simulink model "testbench_model_2019a"  (R2019a)
settings: Solver=ode15s  StartTime=0.0  StopTime=tsim  RelTol=1e-3  EnableMultiTasking=on
values from neighbouring files (symbols this model uses):
  a = randn(1,5)    [magnetic_dist_noise.m]    (also in matlab.mat = 1000)
  g = 9.81    [matlab.mat]    (also in system_dynamics.m = evalin('base','g'))
  Kd1 = 55255.4666667    [matlab.mat]
  Kd3 = 22055.4666667    [matlab.mat]
  Kd4 = 0.01059999556    [matlab.mat]
  Ki1 = 1786382.33784    [matlab.mat]
  Ki3 = 714981.495471    [matlab.mat]
  Ki4 = 13.0608621147    [matlab.mat]
  Kp1 = 551410.490045    [matlab.mat]
  Kp3 = 220696.481621    [matlab.mat]
  Kp4 = 0.623941757147    [matlab.mat]
  mb = 0.2    [matlab.mat]    (also in system_dynamics.m = evalin('base','mb'))
  mj3 = 200    [matlab.mat]    (also in system_dynamics.m = evalin('base','mj3'))
  Tsampling = 0.01    [matlab.mat]
libraries: simulink x9, aerolibnav x2
settings Model: Creator=Akos  LastModifiedBy=akosodry
settings DataIOCC: LimitDataPoints=on  SaveFormat=Array  ReturnWorkspaceOutputs=off
settings OptimizationCC: LifeSpan=inf
settings DebuggingCC: SFUnexpectedBacktrackingDiag=warning  SFNoUnconditionalDefaultTransitionDiag=warning  SFExecutionAtInitializationDiag=none  ArithmeticOperatorsInVariantConditions=warning
settings HardwareCC: ProdBitPerPointer=32  ProdBitPerSizeT=32  ProdBitPerPtrDiffT=32  ProdLargestAtomicFloat=None  ProdIntDivRoundTo=Undefined  ProdEndianess=Unspecified  ProdWordSize=32  ProdHWDeviceType=32-bit Generic
settings ModelReferenceCC: PropagateSignalLabelsOutOfModel=off
settings SFSimCC: SimUseLocalCustomCode=off
settings RTWCC: RTWUseLocalCustomCode=off
settings CodeAppCC: StateflowObjectComments=on
settings GRTTargetCC: TargetLangStandard=C89/C90 (ANSI)  GeneratePreprocessorConditionals=Disable all
settings ConfigComp: CovMetricSettings=dw  CovHtmlReporting=on  CovSaveCumulativeToWorkspaceVar=on  CovSaveSingleToWorkspaceVar=on  CovExternalEMLEnable=off

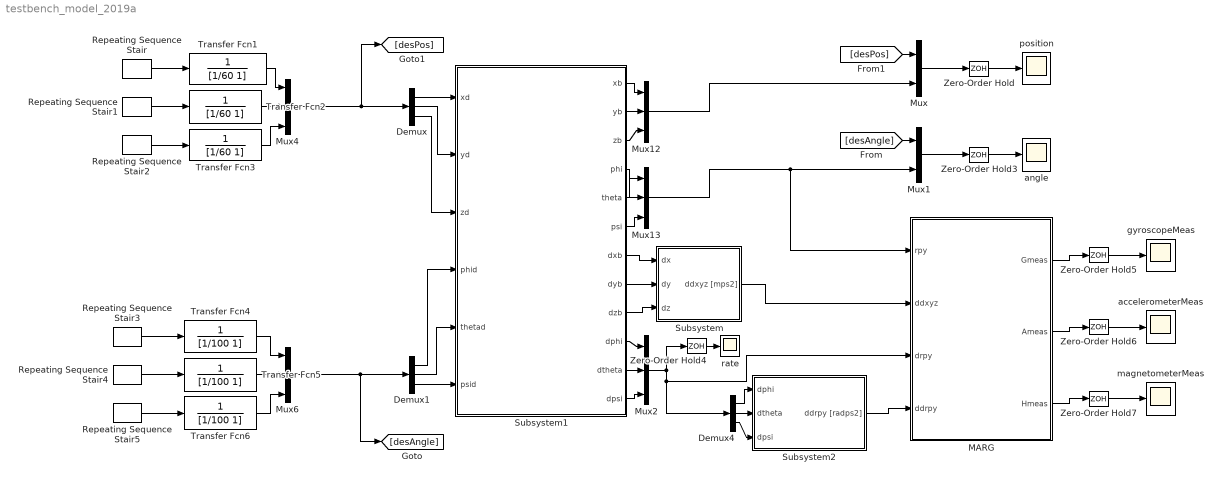
== system testbench_model_2019a ==
  Demux : Demux  Outputs=3
  Demux1 : Demux  Outputs=3
  Demux4 : Demux  Outputs=3
  MARG : Subsystem
  Mux : Mux  Inputs=2
  Mux1 : Mux  Inputs=2
  Mux{2,4,6,12..13} (5 alike) : Mux  Inputs=3
  Repeating Sequence Stair : simulink/Sources/Repeating Sequence Stair  OutValues=[0.5 0.4 0.5 0.1 0.05 0.1 0.9 0.8 0.9].'  tsamp=0.25  OutMin=[]  OutMax=[]  OutDataTypeStr=double  OutputDataTypeScalingMode=double  OutDataType=fixdt(0,8)  ConRadixGroup=Best Precision: Vector-wise  OutScaling=2^-12
  Repeating Sequence Stair1 : simulink/Sources/Repeating Sequence Stair  OutValues=[0.2 0.3 0.2 0.8 0.7 0.8 0.4 0.5 0.4].'  tsamp=0.25  OutMin=[]  OutMax=[]  OutDataTypeStr=double  OutputDataTypeScalingMode=double  OutDataType=fixdt(0,8)  ConRadixGroup=Best Precision: Vector-wise  OutScaling=2^-12
  Repeating Sequence Stair2 : simulink/Sources/Repeating Sequence Stair  OutValues=[0.3 0.2 0.3 0 0.1 0 0.51 0.61 0.51].'  tsamp=0.25  OutMin=[]  OutMax=[]  OutDataTypeStr=double  OutputDataTypeScalingMode=double  OutDataType=fixdt(0,8)  ConRadixGroup=Best Precision: Vector-wise  OutScaling=2^-12
  Repeating Sequence Stair3 : simulink/Sources/Repeating Sequence Stair  OutValues=[0 0.1 0 0.75 0.85 0.75 -0.57 -0.47 -0.57].'  tsamp=0.25  OutMin=[]  OutMax=[]  OutDataTypeStr=double  OutputDataTypeScalingMode=double  OutDataType=fixdt(0,8)  ConRadixGroup=Best Precision: Vector-wise  OutScaling=2^-12
  Repeating Sequence Stair4 : simulink/Sources/Repeating Sequence Stair  OutValues=[0 -0.1 0 0.75 0.65 0.75 -0.19 -0.29 -0.19].'  tsamp=0.25  OutMin=[]  OutMax=[]  OutDataTypeStr=double  OutputDataTypeScalingMode=double  OutDataType=fixdt(0,8)  ConRadixGroup=Best Precision: Vector-wise  OutScaling=2^-12
  Repeating Sequence Stair5 : simulink/Sources/Repeating Sequence Stair  OutValues=[0 0.1 0.1 0.75 0.6 0.75 0.38 0.5 0.38].'  tsamp=0.25  OutMin=[]  OutMax=[]  OutDataTypeStr=double  OutputDataTypeScalingMode=double  OutDataType=fixdt(0,8)  ConRadixGroup=Best Precision: Vector-wise  OutScaling=2^-12
  Subsystem : Subsystem
  Subsystem1 : Subsystem
  Subsystem2 : Subsystem
  Transfer Fcn1 : TransferFcn  Denominator=[1/60 1]
  Transfer Fcn2 : TransferFcn  Denominator=[1/60 1]
  Transfer Fcn3 : TransferFcn  Denominator=[1/60 1]
  Transfer Fcn4 : TransferFcn  Denominator=[1/100 1]
  Transfer Fcn5 : TransferFcn  Denominator=[1/100 1]
  Transfer Fcn6 : TransferFcn  Denominator=[1/100 1]
  Zero-Order Hold{,3..7} (6 alike) : ZeroOrderHold  SampleTime=Tsampling
  accelerometerMeas : Scope
  angle : Scope
  gyroscopeMeas : Scope
  magnetometerMeas : Scope
  position : Scope
  rate : Scope
  wires:
  Mux/1 -> Zero-Order Hold/1
  Mux2/1 -> Demux4/1, MARG/3(drpy), Zero-Order Hold4/1
  Subsystem1/7(dxb) -> Subsystem/1(dx)
  Subsystem1/8(dyb) -> Subsystem/2(dy)
  Subsystem1/9(dzb) -> Subsystem/3(dz)
  Subsystem1/10(dphi) -> Mux2/1
  Subsystem1/11(dtheta) -> Mux2/2
  Subsystem1/12(dpsi) -> Mux2/3
  Repeating Sequence Stair1/1 -> Transfer Fcn2/1
  Repeating Sequence Stair/1 -> Transfer Fcn1/1
  Repeating Sequence Stair2/1 -> Transfer Fcn3/1
  Mux4/1 -> [desPos], Demux/1
  Demux/1 -> Subsystem1/1(xd)
  Demux/2 -> Subsystem1/2(yd)
  Demux/3 -> Subsystem1/3(zd)
  Mux6/1 -> [desAngle], Demux1/1
  Demux1/3 -> Subsystem1/6(psid)
  Demux1/2 -> Subsystem1/5(thetad)
  Demux1/1 -> Subsystem1/4(phid)
  [desAngle] -> Mux1/1
  [desPos] -> Mux/1
  Repeating Sequence Stair4/1 -> Transfer Fcn5/1
  Repeating Sequence Stair3/1 -> Transfer Fcn4/1
  Repeating Sequence Stair5/1 -> Transfer Fcn6/1
  Mux1/1 -> Zero-Order Hold3/1
  Zero-Order Hold/1 -> position/1
  Zero-Order Hold3/1 -> angle/1
  Zero-Order Hold4/1 -> rate/1
  Subsystem1/2(yb) -> Mux12/2
  Subsystem1/3(zb) -> Mux12/3
  Subsystem1/1(xb) -> Mux12/1
  Mux12/1 -> Mux/2
  Subsystem1/4(phi) -> Mux13/1
  Subsystem1/5(theta) -> Mux13/2
  Subsystem1/6(psi) -> Mux13/3
  Mux13/1 -> MARG/1(rpy), Mux1/2
  Demux4/2 -> Subsystem2/2(dtheta)
  Demux4/1 -> Subsystem2/1(dphi)
  Demux4/3 -> Subsystem2/3(dpsi)
  Subsystem/1(ddxyz [mps2]) -> MARG/2(ddxyz)
  Subsystem2/1(ddrpy [radps2]) -> MARG/4(ddrpy)
  MARG/1(Gmeas) -> Zero-Order Hold5/1
  MARG/2(Ameas) -> Zero-Order Hold6/1
  MARG/3(Hmeas) -> Zero-Order Hold7/1
  Transfer Fcn1/1 -> Mux4/1
  Transfer Fcn2/1 -> Mux4/2
  Transfer Fcn3/1 -> Mux4/3
  Transfer Fcn4/1 -> Mux6/1
  Transfer Fcn5/1 -> Mux6/2
  Transfer Fcn6/1 -> Mux6/3
  Zero-Order Hold5/1 -> gyroscopeMeas/1
  Zero-Order Hold6/1 -> accelerometerMeas/1
  Zero-Order Hold7/1 -> magnetometerMeas/1

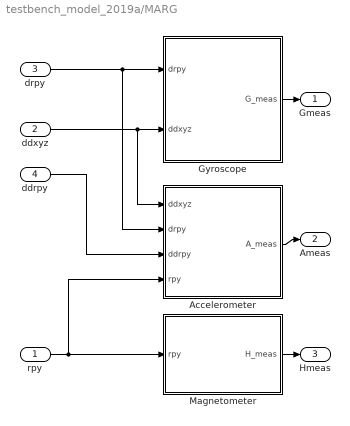
== system testbench_model_2019a/MARG ==
  rpy : Inport
  ddxyz : Inport  Port=2
  drpy : Inport  Port=3
  ddrpy : Inport  Port=4
  Accelerometer : Subsystem
  Gyroscope : Subsystem
  Magnetometer : Subsystem
  Gmeas : Outport
  Ameas : Outport  Port=2
  Hmeas : Outport  Port=3
  wires:
  Magnetometer/1(H_meas) -> Hmeas/1
  Accelerometer/1(A_meas) -> Ameas/1
  Gyroscope/1(G_meas) -> Gmeas/1
  drpy/1 -> Accelerometer/2(drpy), Gyroscope/1(drpy)
  ddrpy/1 -> Accelerometer/3(ddrpy)
  rpy/1 -> Accelerometer/4(rpy), Magnetometer/1(rpy)
  ddxyz/1 -> Gyroscope/2(ddxyz), Accelerometer/1(ddxyz)

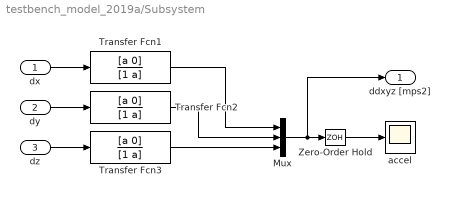
== system testbench_model_2019a/Subsystem ==
  dx : Inport
  dy : Inport  Port=2
  dz : Inport  Port=3
  Mux : Mux  Inputs=3
  Transfer Fcn1 : TransferFcn  Numerator=[a 0]  Denominator=[1 a]
  Transfer Fcn2 : TransferFcn  Numerator=[a 0]  Denominator=[1 a]
  Transfer Fcn3 : TransferFcn  Numerator=[a 0]  Denominator=[1 a]
  Zero-Order Hold : ZeroOrderHold  SampleTime=Tsampling
  accel : Scope
  ddxyz [mps2] : Outport
  wires:
  dz/1 -> Transfer Fcn3/1
  dx/1 -> Transfer Fcn1/1
  dy/1 -> Transfer Fcn2/1
  Transfer Fcn1/1 -> Mux/1
  Mux/1 -> ddxyz [mps2]/1, Zero-Order Hold/1
  Transfer Fcn2/1 -> Mux/2
  Transfer Fcn3/1 -> Mux/3
  Zero-Order Hold/1 -> accel/1

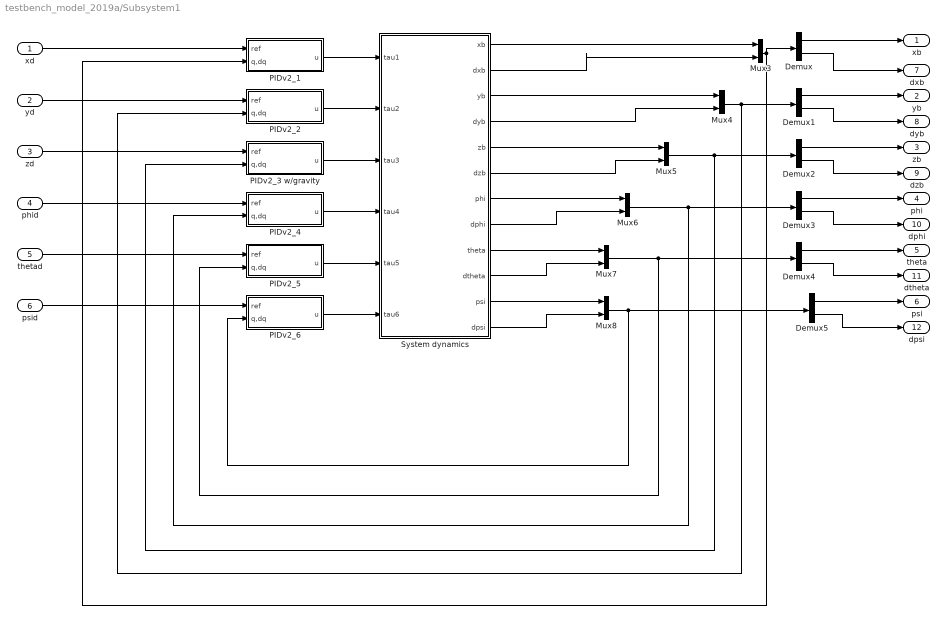
== system testbench_model_2019a/Subsystem1 ==
  xd : Inport
  yd : Inport  Port=2
  zd : Inport  Port=3
  phid : Inport  Port=4
  thetad : Inport  Port=5
  psid : Inport  Port=6
  Demux{,1..5} (6 alike) : Demux  Outputs=2
  Mux{3..8} (6 alike) : Mux  Inputs=2
  PIDv2_1 : Subsystem
  PIDv2_2 : Subsystem
  PIDv2_3 w/gravity : Subsystem
  PIDv2_4 : Subsystem
  PIDv2_5 : Subsystem
  PIDv2_6 : Subsystem
  System dynamics : Subsystem
  xb : Outport
  yb : Outport  Port=2
  zb : Outport  Port=3
  phi : Outport  Port=4
  theta : Outport  Port=5
  psi : Outport  Port=6
  dxb : Outport  Port=7
  dyb : Outport  Port=8
  dzb : Outport  Port=9
  dphi : Outport  Port=10
  dtheta : Outport  Port=11
  dpsi : Outport  Port=12
  wires:
  PIDv2_5/1(u) -> System dynamics/5(tau5)
  Mux3/1 -> Demux/1, PIDv2_1/2(q,dq)
  Demux1/2 -> dyb/1
  Mux8/1 -> Demux5/1, PIDv2_6/2(q,dq)
  Demux4/1 -> theta/1
  psid/1 -> PIDv2_6/1(ref)
  yd/1 -> PIDv2_2/1(ref)
  Mux5/1 -> Demux2/1, PIDv2_3 w/gravity/2(q,dq)
  Demux2/2 -> dzb/1
  xd/1 -> PIDv2_1/1(ref)
  Demux3/1 -> phi/1
  PIDv2_2/1(u) -> System dynamics/2(tau2)
  System dynamics/9(theta) -> Mux7/1
  Demux/1 -> xb/1
  Mux4/1 -> Demux1/1, PIDv2_2/2(q,dq)
  Demux/2 -> dxb/1
  Demux5/2 -> dpsi/1
  System dynamics/12(dpsi) -> Mux8/2
  Mux7/1 -> Demux4/1, PIDv2_5/2(q,dq)
  Mux6/1 -> Demux3/1, PIDv2_4/2(q,dq)
  Demux3/2 -> dphi/1
  phid/1 -> PIDv2_4/1(ref)
  System dynamics/8(dphi) -> Mux6/2
  Demux2/1 -> zb/1
  PIDv2_1/1(u) -> System dynamics/1(tau1)
  Demux1/1 -> yb/1
  System dynamics/3(yb) -> Mux4/1
  PIDv2_4/1(u) -> System dynamics/4(tau4)
  System dynamics/7(phi) -> Mux6/1
  System dynamics/1(xb) -> Mux3/1
  System dynamics/10(dtheta) -> Mux7/2
  System dynamics/6(dzb) -> Mux5/2
  System dynamics/11(psi) -> Mux8/1
  Demux4/2 -> dtheta/1
  PIDv2_6/1(u) -> System dynamics/6(tau6)
  Demux5/1 -> psi/1
  zd/1 -> PIDv2_3 w/gravity/1(ref)
  System dynamics/2(dxb) -> Mux3/2
  System dynamics/4(dyb) -> Mux4/2
  thetad/1 -> PIDv2_5/1(ref)
  PIDv2_3 w/gravity/1(u) -> System dynamics/3(tau3)
  System dynamics/5(zb) -> Mux5/1

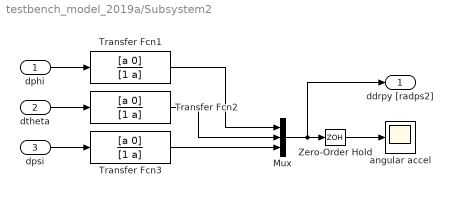
== system testbench_model_2019a/Subsystem2 ==
  dphi : Inport
  dtheta : Inport  Port=2
  dpsi : Inport  Port=3
  Mux : Mux  Inputs=3
  Transfer Fcn1 : TransferFcn  Numerator=[a 0]  Denominator=[1 a]
  Transfer Fcn2 : TransferFcn  Numerator=[a 0]  Denominator=[1 a]
  Transfer Fcn3 : TransferFcn  Numerator=[a 0]  Denominator=[1 a]
  Zero-Order Hold : ZeroOrderHold  SampleTime=Tsampling
  angular accel : Scope
  ddrpy [radps2] : Outport
  wires:
  dpsi/1 -> Transfer Fcn3/1
  dphi/1 -> Transfer Fcn1/1
  dtheta/1 -> Transfer Fcn2/1
  Transfer Fcn1/1 -> Mux/1
  Mux/1 -> ddrpy [radps2]/1, Zero-Order Hold/1
  Transfer Fcn2/1 -> Mux/2
  Transfer Fcn3/1 -> Mux/3
  Zero-Order Hold/1 -> angular accel/1

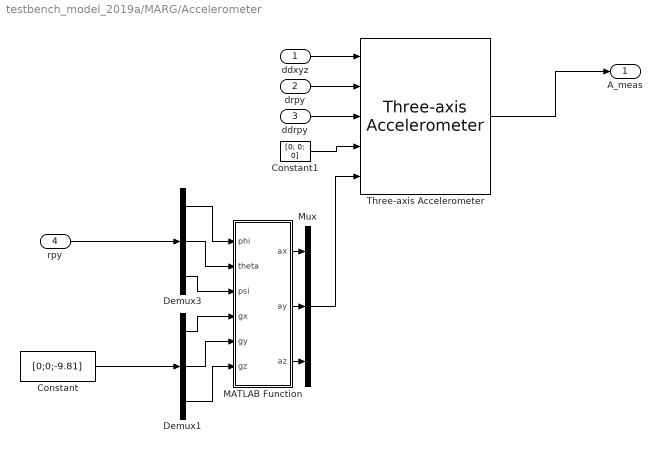
== system testbench_model_2019a/MARG/Accelerometer ==
  ddxyz : Inport
  drpy : Inport  Port=2
  ddrpy : Inport  Port=3
  rpy : Inport  Port=4
  Constant : Constant  Value=[0;0;-9.81]
  Constant1 : Constant  Value=[0; 0; 0]
  Demux1 : Demux  Outputs=3
  Demux3 : Demux  Outputs=3
  MATLAB Function : MATLAB Function  TreatAsAtomicUnit=on
  Mux : Mux  Inputs=3
  Three-axis Accelerometer : aerolibnav/Three-axis Accelerometer  units=Metric (MKS)  acc=[0 0 0]  gtype=on  dtype_a=off  w_a=190  z_a=0.707  a_sf_cc=[1 0 0; 0 1 0; 0 0 1]  a_bias=[0 0 0]  a_Ts=Tsampling  a_rand=on  a_seeds=[23093 23094 23095]  a_pow=[0.0005 0.0005 0.0005]  a_sat="[-inf  -inf  -inf  inf inf inf]"
      settings: SourceProductName=Aerospace Blockset  SourceProductBaseCode=AE
  A_meas : Outport
  wires:
  Three-axis Accelerometer/1 -> A_meas/1
  ddxyz/1 -> Three-axis Accelerometer/1
  Demux1/2 -> MATLAB Function/5(gy)
  Demux3/1 -> MATLAB Function/1(phi)
  Demux3/2 -> MATLAB Function/2(theta)
  MATLAB Function/2(ay) -> Mux/2
  Demux3/3 -> MATLAB Function/3(psi)
  Demux1/3 -> MATLAB Function/6(gz)
  MATLAB Function/1(ax) -> Mux/1
  MATLAB Function/3(az) -> Mux/3
  Demux1/1 -> MATLAB Function/4(gx)
  rpy/1 -> Demux3/1
  Constant/1 -> Demux1/1
  Mux/1 -> Three-axis Accelerometer/5
  drpy/1 -> Three-axis Accelerometer/2
  ddrpy/1 -> Three-axis Accelerometer/3
  Constant1/1 -> Three-axis Accelerometer/4

== system testbench_model_2019a/MARG/Gyroscope ==
  drpy : Inport
  ddxyz : Inport  Port=2
  Gain2 : Gain  Gain=1/g
  Three-axis Gyroscope : aerolibnav/Three-axis Gyroscope  dtype_g=on  w_g=190  z_g=0.707  g_sf_cc=[1 0 0; 0 1 0; 0 0 1]  g_bias=[0 0 0]  g_sen=[0 0 0]  g_Ts=Tsampling  g_rand=on  g_seeds=[23093 23094 23095]  g_pow=[0.0005 0.0005 0.0005]  g_sat="[-inf  -inf  -inf  inf inf inf]"
      settings: SourceProductName=Aerospace Blockset  SourceProductBaseCode=AE
  G_meas : Outport
  wires:
  ddxyz/1 -> Gain2/1
  Gain2/1 -> Three-axis Gyroscope/2
  Three-axis Gyroscope/1 -> G_meas/1
  drpy/1 -> Three-axis Gyroscope/1

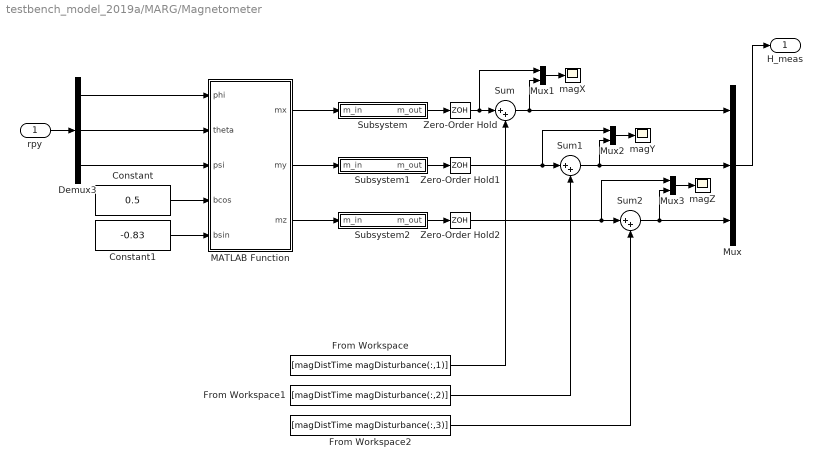
== system testbench_model_2019a/MARG/Magnetometer ==
  rpy : Inport
  Constant : Constant  Value=0.5
  Constant1 : Constant  Value=-0.83
  Demux3 : Demux  Outputs=3
  From Workspace : FromWorkspace  VariableName=[magDistTime magDisturbance(:,1)]  SampleTime=Tsampling
  From Workspace1 : FromWorkspace  VariableName=[magDistTime magDisturbance(:,2)]  SampleTime=Tsampling
  From Workspace2 : FromWorkspace  VariableName=[magDistTime magDisturbance(:,3)]  SampleTime=Tsampling
  MATLAB Function : MATLAB Function  TreatAsAtomicUnit=on
  Mux : Mux  Inputs=3
  Mux1 : Mux  Inputs=2
  Mux2 : Mux  Inputs=2
  Mux3 : Mux  Inputs=2
  Subsystem : Subsystem
  Subsystem1 : Subsystem
  Subsystem2 : Subsystem
  Sum : Sum  Inputs=|++
  Sum1 : Sum  Inputs=|++
  Sum2 : Sum  Inputs=|++
  Zero-Order Hold : ZeroOrderHold  SampleTime=Tsampling
  Zero-Order Hold1 : ZeroOrderHold  SampleTime=Tsampling
  Zero-Order Hold2 : ZeroOrderHold  SampleTime=Tsampling
  magX : Scope
  magY : Scope
  magZ : Scope
  H_meas : Outport
  wires:
  Demux3/3 -> MATLAB Function/3(psi)
  Demux3/1 -> MATLAB Function/1(phi)
  Mux/1 -> H_meas/1
  Constant/1 -> MATLAB Function/4(bcos)
  Constant1/1 -> MATLAB Function/5(bsin)
  MATLAB Function/1(mx) -> Subsystem/1(m_in)
  Subsystem/1(m_out) -> Zero-Order Hold/1
  rpy/1 -> Demux3/1
  Demux3/2 -> MATLAB Function/2(theta)
  MATLAB Function/2(my) -> Subsystem1/1(m_in)
  Subsystem1/1(m_out) -> Zero-Order Hold1/1
  MATLAB Function/3(mz) -> Subsystem2/1(m_in)
  Subsystem2/1(m_out) -> Zero-Order Hold2/1
  Zero-Order Hold/1 -> Mux1/1, Sum/1
  Sum/1 -> Mux1/2, Mux/1
  Zero-Order Hold1/1 -> Mux2/1, Sum1/1
  Sum1/1 -> Mux2/2, Mux/2
  From Workspace/1 -> Sum/2
  Mux1/1 -> magX/1
  From Workspace1/1 -> Sum1/2
  Mux2/1 -> magY/1
  Mux3/1 -> magZ/1
  Sum2/1 -> Mux3/2, Mux/3
  Zero-Order Hold2/1 -> Mux3/1, Sum2/1
  From Workspace2/1 -> Sum2/2

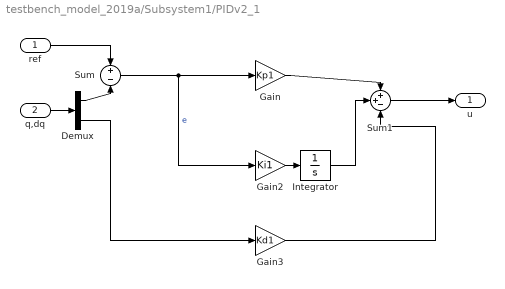
== system testbench_model_2019a/Subsystem1/PIDv2_1 ==
  ref : Inport
  q,dq : Inport  Port=2
  Demux : Demux  Outputs=2
  Gain : Gain  Gain=Kp1
  Gain2 : Gain  Gain=Ki1
  Gain3 : Gain  Gain=Kd1
  Integrator : Integrator
  Sum : Sum  Inputs=+-
  Sum1 : Sum  Inputs=++-
  u : Outport
  wires:
  Sum1/1 -> u/1
  Gain3/1 -> Sum1/3
  Demux/1 -> Sum/2
  Gain2/1 -> Integrator/1
  Gain/1 -> Sum1/1
  Integrator/1 -> Sum1/2
  Demux/2 -> Gain3/1
  q,dq/1 -> Demux/1
  ref/1 -> Sum/1
  Sum/1 -> Gain2/1, Gain/1  "e"

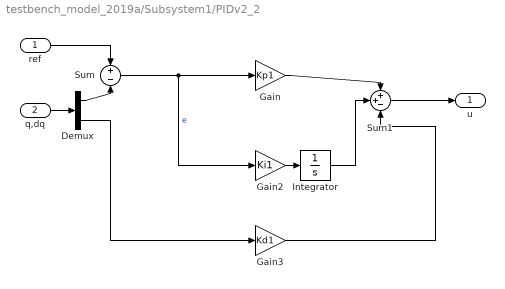
== system testbench_model_2019a/Subsystem1/PIDv2_2 ==
  ref : Inport
  q,dq : Inport  Port=2
  Demux : Demux  Outputs=2
  Gain : Gain  Gain=Kp1
  Gain2 : Gain  Gain=Ki1
  Gain3 : Gain  Gain=Kd1
  Integrator : Integrator
  Sum : Sum  Inputs=+-
  Sum1 : Sum  Inputs=++-
  u : Outport
  wires:
  Sum1/1 -> u/1
  Gain3/1 -> Sum1/3
  Demux/1 -> Sum/2
  Gain2/1 -> Integrator/1
  Gain/1 -> Sum1/1
  Integrator/1 -> Sum1/2
  Demux/2 -> Gain3/1
  q,dq/1 -> Demux/1
  ref/1 -> Sum/1
  Sum/1 -> Gain2/1, Gain/1  "e"

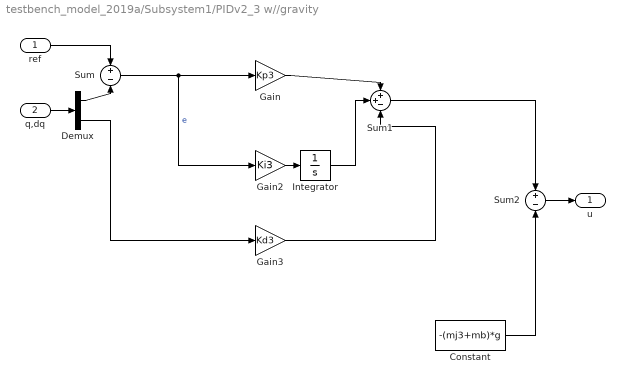
== system testbench_model_2019a/Subsystem1/PIDv2_3 w//gravity ==
  ref : Inport
  q,dq : Inport  Port=2
  Constant : Constant  Value=-(mj3+mb)*g
  Demux : Demux  Outputs=2
  Gain : Gain  Gain=Kp3
  Gain2 : Gain  Gain=Ki3
  Gain3 : Gain  Gain=Kd3
  Integrator : Integrator
  Sum : Sum  Inputs=+-
  Sum1 : Sum  Inputs=++-
  Sum2 : Sum  Inputs=+-
  u : Outport
  wires:
  Gain3/1 -> Sum1/3
  Demux/1 -> Sum/2
  Gain2/1 -> Integrator/1
  Gain/1 -> Sum1/1
  Integrator/1 -> Sum1/2
  Demux/2 -> Gain3/1
  q,dq/1 -> Demux/1
  ref/1 -> Sum/1
  Sum/1 -> Gain2/1, Gain/1  "e"
  Sum1/1 -> Sum2/1
  Constant/1 -> Sum2/2
  Sum2/1 -> u/1

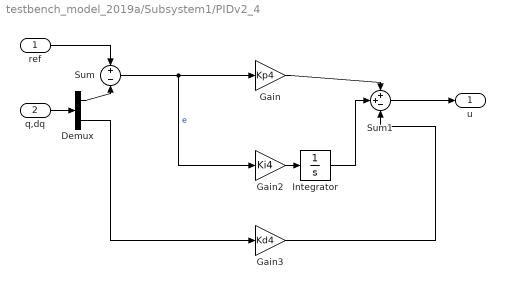
== system testbench_model_2019a/Subsystem1/PIDv2_4 ==
  ref : Inport
  q,dq : Inport  Port=2
  Demux : Demux  Outputs=2
  Gain : Gain  Gain=Kp4
  Gain2 : Gain  Gain=Ki4
  Gain3 : Gain  Gain=Kd4
  Integrator : Integrator
  Sum : Sum  Inputs=+-
  Sum1 : Sum  Inputs=++-
  u : Outport
  wires:
  Sum1/1 -> u/1
  Gain3/1 -> Sum1/3
  Demux/1 -> Sum/2
  Gain2/1 -> Integrator/1
  Gain/1 -> Sum1/1
  Integrator/1 -> Sum1/2
  Demux/2 -> Gain3/1
  q,dq/1 -> Demux/1
  ref/1 -> Sum/1
  Sum/1 -> Gain2/1, Gain/1  "e"

== system testbench_model_2019a/Subsystem1/PIDv2_5 ==
  ref : Inport
  q,dq : Inport  Port=2
  Demux : Demux  Outputs=2
  Gain : Gain  Gain=Kp4
  Gain2 : Gain  Gain=Ki4
  Gain3 : Gain  Gain=Kd4
  Integrator : Integrator
  Sum : Sum  Inputs=+-
  Sum1 : Sum  Inputs=++-
  u : Outport
  wires:
  Sum1/1 -> u/1
  Gain3/1 -> Sum1/3
  Demux/1 -> Sum/2
  Gain2/1 -> Integrator/1
  Gain/1 -> Sum1/1
  Integrator/1 -> Sum1/2
  Demux/2 -> Gain3/1
  q,dq/1 -> Demux/1
  ref/1 -> Sum/1
  Sum/1 -> Gain2/1, Gain/1  "e"

== system testbench_model_2019a/Subsystem1/PIDv2_6 ==
  ref : Inport
  q,dq : Inport  Port=2
  Demux : Demux  Outputs=2
  Gain : Gain  Gain=Kp4
  Gain2 : Gain  Gain=Ki4
  Gain3 : Gain  Gain=Kd4
  Integrator : Integrator
  Sum : Sum  Inputs=+-
  Sum1 : Sum  Inputs=++-
  u : Outport
  wires:
  Sum1/1 -> u/1
  Gain3/1 -> Sum1/3
  Demux/1 -> Sum/2
  Gain2/1 -> Integrator/1
  Gain/1 -> Sum1/1
  Integrator/1 -> Sum1/2
  Demux/2 -> Gain3/1
  q,dq/1 -> Demux/1
  ref/1 -> Sum/1
  Sum/1 -> Gain2/1, Gain/1  "e"

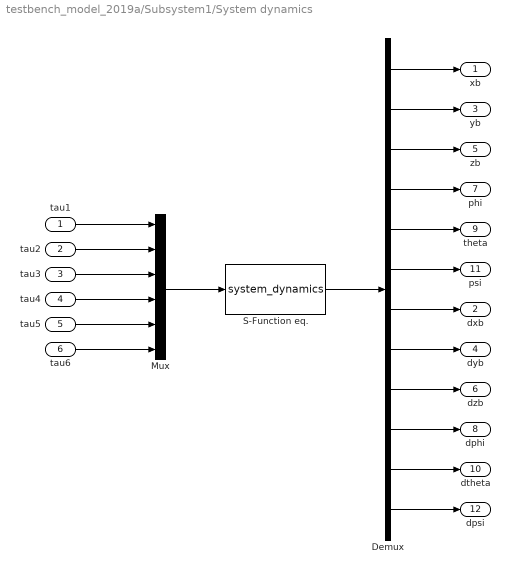
== system testbench_model_2019a/Subsystem1/System dynamics ==
  tau1 : Inport
  tau2 : Inport  Port=2
  tau3 : Inport  Port=3
  tau4 : Inport  Port=4
  tau5 : Inport  Port=5
  tau6 : Inport  Port=6
  Demux : Demux  Outputs=12
  Mux : Mux  Inputs=6
  S-Function eq. : S-Function  FunctionName=system_dynamics  SFunctionDeploymentMode=off  EnableBusSupport=off
  xb : Outport
  dxb : Outport  Port=2
  yb : Outport  Port=3
  dyb : Outport  Port=4
  zb : Outport  Port=5
  dzb : Outport  Port=6
  phi : Outport  Port=7
  dphi : Outport  Port=8
  theta : Outport  Port=9
  dtheta : Outport  Port=10
  psi : Outport  Port=11
  dpsi : Outport  Port=12
  wires:
  Demux/2 -> yb/1
  Demux/1 -> xb/1
  Mux/1 -> S-Function eq./1
  S-Function eq./1 -> Demux/1
  Demux/3 -> zb/1
  tau1/1 -> Mux/1
  tau2/1 -> Mux/2
  tau3/1 -> Mux/3
  tau4/1 -> Mux/4
  tau5/1 -> Mux/5
  tau6/1 -> Mux/6
  Demux/4 -> phi/1
  Demux/5 -> theta/1
  Demux/6 -> psi/1
  Demux/7 -> dxb/1
  Demux/8 -> dyb/1
  Demux/9 -> dzb/1
  Demux/10 -> dphi/1
  Demux/11 -> dtheta/1
  Demux/12 -> dpsi/1

== system testbench_model_2019a/MARG/Magnetometer/Subsystem ==
  m_in : Inport
  Sum : Sum  Inputs=+++
  bias : Constant  Value=0
  dynamics : TransferFcn  Numerator=[(6000)^2]  Denominator=[1 sqrt(2)*6000 (6000)^2]
  noise : simulink/Sources/Band-Limited White Noise  Cov=[0.000005]  Ts=Tsampling  seed=[23341]
  m_out : Outport
  wires:
  m_in/1 -> dynamics/1
  bias/1 -> Sum/2
  dynamics/1 -> Sum/1
  noise/1 -> Sum/3
  Sum/1 -> m_out/1

== system testbench_model_2019a/MARG/Magnetometer/Subsystem1 ==
  m_in : Inport
  Sum : Sum  Inputs=+++
  bias : Constant  Value=0
  dynamics : TransferFcn  Numerator=[(6000)^2]  Denominator=[1 sqrt(2)*6000 (6000)^2]
  noise : simulink/Sources/Band-Limited White Noise  Cov=[0.000005]  Ts=Tsampling  seed=[23341]
  m_out : Outport
  wires:
  m_in/1 -> dynamics/1
  bias/1 -> Sum/2
  dynamics/1 -> Sum/1
  noise/1 -> Sum/3
  Sum/1 -> m_out/1

== system testbench_model_2019a/MARG/Magnetometer/Subsystem2 ==
  m_in : Inport
  Sum : Sum  Inputs=+++
  bias : Constant  Value=0
  dynamics : TransferFcn  Numerator=[(6000)^2]  Denominator=[1 sqrt(2)*6000 (6000)^2]
  noise : simulink/Sources/Band-Limited White Noise  Cov=[0.000005]  Ts=Tsampling  seed=[23341]
  m_out : Outport
  wires:
  m_in/1 -> dynamics/1
  bias/1 -> Sum/2
  dynamics/1 -> Sum/1
  noise/1 -> Sum/3
  Sum/1 -> m_out/1

== matlab function testbench_model_2019a/MARG/Accelerometer/MATLAB Function ==
  data: phi input; ax output; theta input; psi input; ay output; az output; gx input; gy input; gz input
function [ax,ay,az] = fcn(phi, theta, psi, gx, gy, gz)

R = zeros(3,3);
R(1,1) = cos(psi)*cos(theta);
R(1,2) = -sin(psi)*cos(phi) + cos(psi)*sin(theta)*sin(phi);
R(1,3) = sin(psi)*sin(phi) + cos(psi)*sin(theta)*cos(phi);
R(2,1) = sin(psi)*cos(theta);
R(2,2) = cos(psi)*cos(phi) + sin(psi)*sin(theta)*sin(phi);
R(2,3) = -cos(psi)*sin(phi) + sin(psi)*sin(theta)*cos(phi);
R(3,1) = -sin(theta);
R(3,2) = cos(theta)*sin(phi);
R(3,3) = cos(theta)*cos(phi);

m = R'*[gx;gy;gz];

ax = m(1);
ay = m(2);
az = m(3);

== matlab function testbench_model_2019a/MARG/Magnetometer/MATLAB Function ==
  data: phi input; mx output; theta input; psi input; bcos input; bsin input; my output; mz output
function [mx,my,mz] = fcn(phi, theta, psi, bcos, bsin)

R = zeros(3,3);
R(1,1) = cos(psi)*cos(theta);
R(1,2) = -sin(psi)*cos(phi) + cos(psi)*sin(theta)*sin(phi);
R(1,3) = sin(psi)*sin(phi) + cos(psi)*sin(theta)*cos(phi);
R(2,1) = sin(psi)*cos(theta);
R(2,2) = cos(psi)*cos(phi) + sin(psi)*sin(theta)*sin(phi);
R(2,3) = -cos(psi)*sin(phi) + sin(psi)*sin(theta)*cos(phi);
R(3,1) = -sin(theta);
R(3,2) = cos(theta)*sin(phi);
R(3,3) = cos(theta)*cos(phi);

m = R'*[bcos;0;bsin];

mx = m(1);
my = m(2);
mz = m(3);
